simulink model "lab2"  (R2022a)
settings: Solver=VariableStepAuto  StartTime=0.0  StopTime=5.0  RelTol=1e-3
settings Model: Creator=User  LastModifiedBy=User

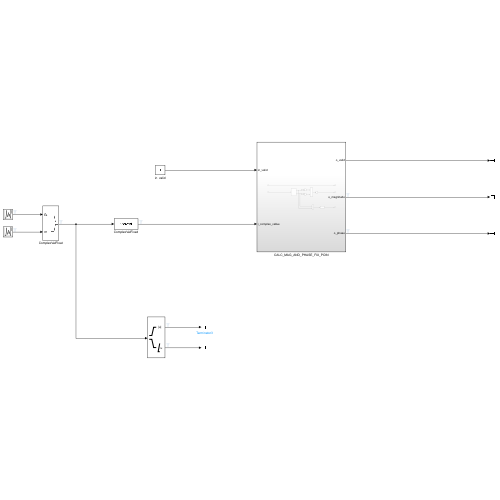
[thumbnail: Simulink's stored preview of the top-level diagram]
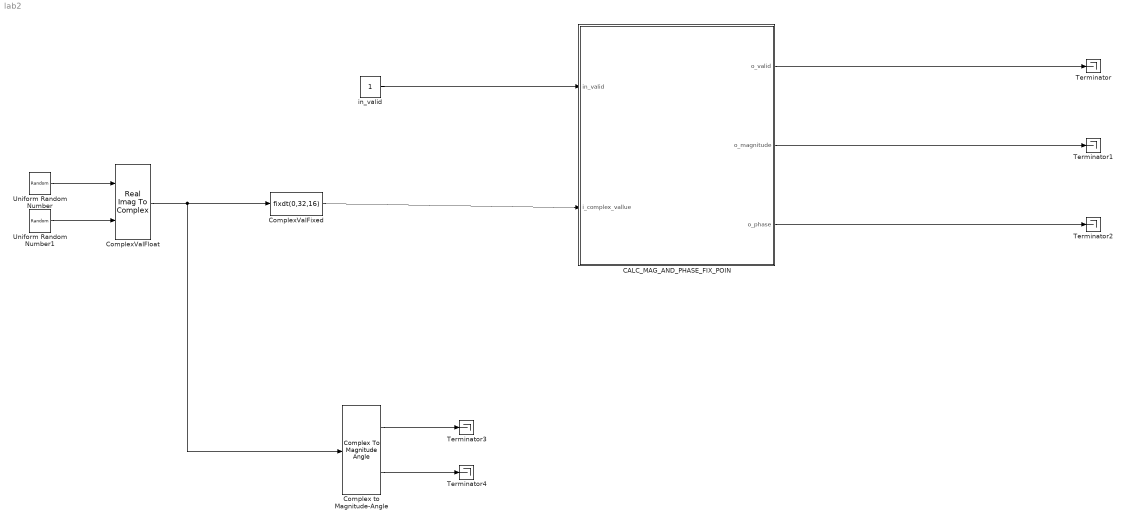
== system lab2 ==
  CALC_MAG_AND_PHASE_FIX_POIN : Subsystem
  Complex to Magnitude-Angle : ComplexToMagnitudeAngle
  ComplexValFixed : DataTypeConversion  OutDataTypeStr=fixdt(0,32,16)  RndMeth=Round  SaturateOnIntegerOverflow=off
  ComplexValFloat : RealImagToComplex
  Terminator{,1..4} (5 alike) : Terminator
  Uniform Random Number : UniformRandomNumber  Minimum=0  Maximum=2 ^(16)-1  Seed=16  SampleTime=1
  Uniform Random Number1 : UniformRandomNumber  Minimum=0  Maximum=2 ^(16)-1  Seed=17  SampleTime=1
  in_valid : Constant  OutDataTypeStr=boolean  SampleTime=1
  wires:
  Uniform Random Number/1 -> ComplexValFloat/1
  Uniform Random Number1/1 -> ComplexValFloat/2
  ComplexValFloat/1 -> Complex to Magnitude-Angle/1, ComplexValFixed/1
  Complex to Magnitude-Angle/1 -> Terminator3/1
  Complex to Magnitude-Angle/2 -> Terminator4/1
  ComplexValFixed/1 -> CALC_MAG_AND_PHASE_FIX_POIN/2(i_complex_vallue)
  CALC_MAG_AND_PHASE_FIX_POIN/2(o_magnitude) -> Terminator1/1
  CALC_MAG_AND_PHASE_FIX_POIN/3(o_phase) -> Terminator2/1
  in_valid/1 -> CALC_MAG_AND_PHASE_FIX_POIN/1(in_valid)
  CALC_MAG_AND_PHASE_FIX_POIN/1(o_valid) -> Terminator/1

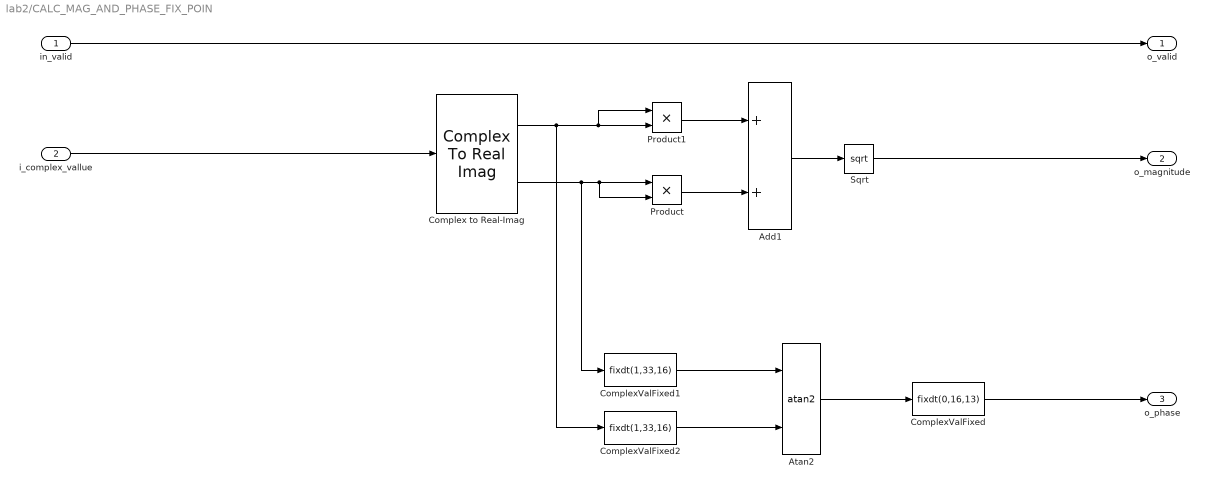
== system lab2/CALC_MAG_AND_PHASE_FIX_POIN ==
  in_valid : Inport  OutDataTypeStr=boolean
  i_complex_vallue : Inport  Port=2
  Add1 : Sum  AccumDataTypeStr=fixdt(0,65,32)  OutDataTypeStr=fixdt(0,65,32)
  Atan2 : Trigonometry  Operator=atan2  ApproximationMethod=CORDIC
  Complex to Real-Imag : ComplexToRealImag
  ComplexValFixed : DataTypeConversion  OutDataTypeStr=fixdt(0,16,13)  RndMeth=Round  SaturateOnIntegerOverflow=off
  ComplexValFixed1 : DataTypeConversion  OutDataTypeStr=fixdt(1,33,16)  RndMeth=Round  SaturateOnIntegerOverflow=off
  ComplexValFixed2 : DataTypeConversion  OutDataTypeStr=fixdt(1,33,16)  RndMeth=Round  SaturateOnIntegerOverflow=off
  Product : Product
  Product1 : Product
  Sqrt : Sqrt  OutDataTypeStr=Inherit: Inherit via internal rule
  o_valid : Outport
  o_magnitude : Outport  Port=2
  o_phase : Outport  Port=3
  wires:
  Complex to Real-Imag/1 -> ComplexValFixed2/1, Product1/1, Product1/2
  Add1/1 -> Sqrt/1
  Complex to Real-Imag/2 -> ComplexValFixed1/1, Product/2, Product/1
  Product1/1 -> Add1/1
  Sqrt/1 -> o_magnitude/1
  Product/1 -> Add1/2
  Atan2/1 -> ComplexValFixed/1
  i_complex_vallue/1 -> Complex to Real-Imag/1
  in_valid/1 -> o_valid/1
  ComplexValFixed/1 -> o_phase/1
  ComplexValFixed1/1 -> Atan2/1
  ComplexValFixed2/1 -> Atan2/2
